simulink model "controllerROS"  (R2021a)
settings: Solver=FixedStepDiscrete  StartTime=0.0  StopTime=200.0  FixedStep=0.02  RelTol=1e-3
undefined symbols (not defined in the file or in its folder): Angular, Linear
libraries: simulink x5, robotlib x3
settings Model: Creator=tian  LastModifiedBy=tian

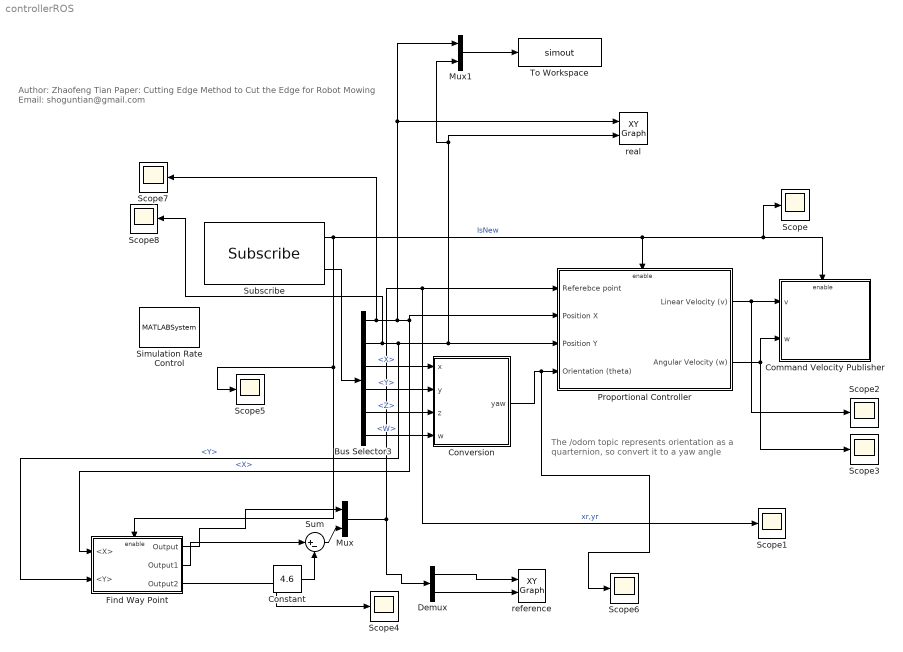
== system controllerROS ==
  note: Author: Zhaofeng Tian
      | Paper: Cutting Edge Method to Cut the Edge for Robot Mowing
      | Email: shoguntian@gmail.com
  note: The /odom topic represents orientation as a quarternion, so convert it to a yaw angle
  Bus Selector3 : BusSelector  OutputSignals=Pose.Pose.Position.X,Pose.Pose.Position.Y,Pose.Pose.Orientation.X,Pose.Pose.Orientation.Y,Pose.Pose.Orientation.Z,Pose.Pose.Orientation.W
  Command Velocity Publisher : Subsystem
  Constant : Constant  Value=4.6
  Conversion : MATLAB Function  TreatAsAtomicUnit=on
  Demux : Demux  Outputs=2
  Find Way Point : Subsystem
  Mux : Mux  Inputs=2
  Mux1 : Mux  Inputs=2
  Proportional Controller : Subsystem
  Scope{,1..8} (9 alike) : Scope
  Simulation Rate Control : MATLABSystem  System=ExampleHelperSimulationRateControl  SampleTime=0.02
      mask Type: ExampleHelperSimulationRateControl
      mask Display: disp('Rate Control');
  Subscribe : robotlib/Subscribe  topicSource=Select from ROS network  topic=/odom  messageType=nav_msgs/Odometry  SampleTime=-1  legacyBusStruct=off  messageQueueLength=51
  Sum : Sum  Inputs=|+-
  To Workspace : ToWorkspace  VariableName=simout  SaveFormat=Timeseries  SampleTime=-1
  real : simulink/Sinks/XY Graph  xmin=-1  xmax=11  ymin=-5  ymax=5  st=-1
  "reference " : simulink/Sinks/XY Graph  xmin=-1  xmax=11  ymin=-5  ymax=5  st=-1
  wires:
  Bus Selector3/2 -> Scope8/1, Find Way Point/2(<Y>), Mux1/2, real/2, Proportional Controller/3(Position Y)  "<Y>"
  Bus Selector3/4 -> Conversion/2(y)  "<Y>"
  Subscribe/1 -> Scope5/1, Find Way Point/Enable, Command Velocity Publisher/Enable, Scope/1, Proportional Controller/Enable  "IsNew"
  Proportional Controller/1(Linear Velocity (v)) -> Scope2/1, Command Velocity Publisher/1(v)
  Bus Selector3/6 -> Conversion/4(w)  "<W>"
  Bus Selector3/1 -> Mux1/1, real/1, Find Way Point/1(<X>), Proportional Controller/2(Position X), Scope7/1  "<X>"
  Mux/1 -> Proportional Controller/1(Referebce point), Scope1/1, Demux/1  "xr,yr"
  Conversion/1(yaw) -> Scope6/1, Proportional Controller/4(Orientation (theta))
  Bus Selector3/5 -> Conversion/3(z)  "<Z>"
  Bus Selector3/3 -> Conversion/1(x)  "<X>"
  Subscribe/2 -> Bus Selector3/1
  Proportional Controller/2(Angular Velocity (w)) -> Command Velocity Publisher/2(w), Scope3/1
  Demux/1 -> "reference "/1
  Demux/2 -> "reference "/2
  Find Way Point/1(Output) -> Mux/1
  Find Way Point/3(Output2) -> Scope4/1
  Mux1/1 -> To Workspace/1
  Find Way Point/2(Output1) -> Sum/1
  Constant/1 -> Sum/2
  Sum/1 -> Mux/2

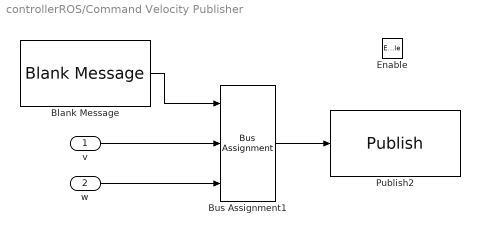
== system controllerROS/Command Velocity Publisher ==
  v : Inport
  w : Inport  Port=2
  Enable : EnablePort
  Blank Message : robotlib/Blank Message  messageClass=Message  entityType=geometry_msgs/Twist  messageType=geometry_msgs/Twist  SampleTime=inf  legacyBusStruct=off
  Bus Assignment1 : BusAssignment  DialogController=Simulink.DDGSource_BusAssignment  AssignedSignals=Linear.X,Angular.Z
  Publish2 : robotlib/Publish  topicSource=Select from ROS network  topic=/cmd_vel  messageType=geometry_msgs/Twist  legacyBusStruct=off  messageQueueLength=105
  wires:
  Bus Assignment1/1 -> Publish2/1
  Blank Message/1 -> Bus Assignment1/1
  v/1 -> Bus Assignment1/2
  w/1 -> Bus Assignment1/3

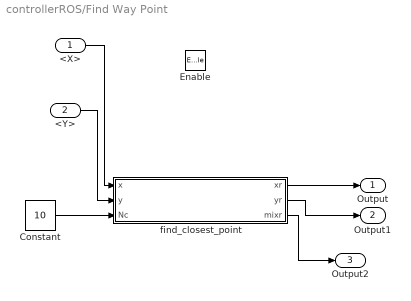
== system controllerROS/Find Way Point ==
  <X> : Inport
  <Y> : Inport  Port=2
  Enable : EnablePort
  Constant : Constant  Value=10
  find_closest_point : MATLAB Function  TreatAsAtomicUnit=on
  Output : Outport
  Output1 : Outport  Port=2
  Output2 : Outport  Port=3
  wires:
  find_closest_point/3(mixr) -> Output2/1
  find_closest_point/2(yr) -> Output1/1
  find_closest_point/1(xr) -> Output/1
  <X>/1 -> find_closest_point/1(x)
  Constant/1 -> find_closest_point/3(Nc)
  <Y>/1 -> find_closest_point/2(y)

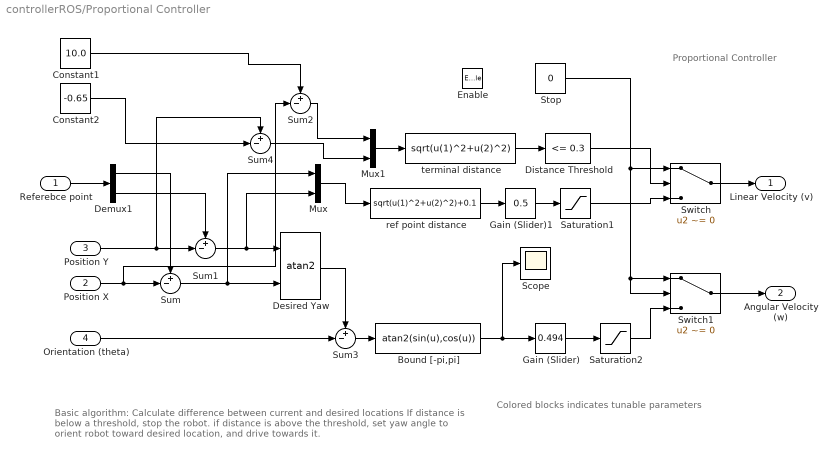
== system controllerROS/Proportional Controller ==
  note: Proportional Controller
  note: Basic algorithm:
      | Calculate difference between current and desired locations
      | If distance is below a threshold, stop the robot.
      | if distance is above the threshold, set yaw angle to orient robot toward desired location, and drive towards it.
  note: Colored blocks indicates tunable parameters
  Referebce point : Inport
  Position X : Inport  Port=2
  Position Y : Inport  Port=3
  Orientation (theta) : Inport  Port=4
  Enable : EnablePort
  Bound [-pi,pi] : Fcn  Expr=atan2(sin(u),cos(u))
  Constant1 : Constant  Value=10.0
  Constant2 : Constant  Value=-0.65
  Demux1 : Demux  Outputs=2
  Desired Yaw : Trigonometry  Operator=atan2
  Distance Threshold : simulink/Logic and Bit Operations/Compare To Constant  relop=<=  const=0.3  OutDataTypeStr=boolean
  Gain (Slider) : simulink/Math Operations/Slider Gain  gain=0.494  low=0.2  high=10
  Gain (Slider)1 : simulink/Math Operations/Slider Gain  gain=0.5  low=0.2  high=10
  Mux : Mux  Inputs=2
  Mux1 : Mux  Inputs=2
  Saturation1 : Saturate  UpperLimit=0.2  LowerLimit=-0.2
  Saturation2 : Saturate  UpperLimit=0.4  LowerLimit=-0.4
  Scope : Scope
  Stop : Constant  Value=0
  Sum{,1..4} (5 alike) : Sum  Inputs=+-|
  Switch : Switch  Criteria=u2 ~= 0
  Switch1 : Switch  Criteria=u2 ~= 0
  ref point distance : Fcn  Expr=sqrt(u(1)^2+u(2)^2)+0.1
  terminal distance : Fcn  Expr=sqrt(u(1)^2+u(2)^2)
  Linear Velocity (v) : Outport  VectorParamsAs1DForOutWhenUnconnected=off
  Angular Velocity (w) : Outport  Port=2  VectorParamsAs1DForOutWhenUnconnected=off
  wires:
  Demux1/1 -> Sum/1
  Demux1/2 -> Sum1/1
  Sum1/1 -> Desired Yaw/1, Mux/2
  Referebce point/1 -> Demux1/1
  Position Y/1 -> Sum4/1, Sum1/2
  Position X/1 -> Sum2/2, Sum/2
  Mux/1 -> ref point distance/1
  Bound [-pi,pi]/1 -> Scope/1, Gain (Slider)/1
  Orientation (theta)/1 -> Sum3/2
  Desired Yaw/1 -> Sum3/1
  Sum/1 -> Desired Yaw/2, Mux/1
  ref point distance/1 -> Gain (Slider)1/1
  Gain (Slider)/1 -> Saturation2/1
  Stop/1 -> Switch/1, Switch1/2, Switch1/1
  Sum3/1 -> Bound [-pi,pi]/1
  Switch/1 -> Linear Velocity (v)/1
  Switch1/1 -> Angular Velocity (w)/1
  Constant1/1 -> Sum2/1
  Constant2/1 -> Sum4/2
  Sum2/1 -> Mux1/1
  Sum4/1 -> Mux1/2
  Mux1/1 -> terminal distance/1
  terminal distance/1 -> Distance Threshold/1
  Distance Threshold/1 -> Switch/2
  Saturation1/1 -> Switch/3
  Saturation2/1 -> Switch1/3
  Gain (Slider)1/1 -> Saturation1/1

== matlab function controllerROS/Conversion ==
  data: yaw output; x input; y input; z input; w input
function yaw  = quat2eul(x,y,z,w)
%#codegen

% Convert the quaternion to a yaw angle (zyx euler angle)
eul = quat2eul([w,x,y,z]);
yaw = eul(1);

end

== matlab function controllerROS/Find Way Point/find_closest_point ==
  data: x input; xr output; y input; Nc input; yr output; mixr output
function [xr,yr,mixr]= find_closest_pont(x,y,Nc)
%load planx and plany
mm =load('roadplan.mat');
planx=mm.nnx*mm.dx;
plany=mm.ylist_line_smooth*mm.dy;
plany=plany';

ixr = ceil(x/mm.dx);% dx = 0.01
if ixr <= 0
    ixr = 1;
end
% Initialization
mind = 1000;
mixr = 1;

% Find min distance loop
if ixr <= 1000-Nc
    for i=ixr:ixr+Nc
        tempd=((planx(i)-x)^2+(plany(i)-y)^2)^0.5;
        if tempd < mind
            mind = tempd;% Update min distance
            mixr = i;         % Update min xr index (ixr)
        end
    end
else
    for i=ixr:1000
        tempd=((planx(i)-x)^2+(plany(i)-y)^2)^0.5;
        if tempd < mind
            mind = tempd;
            mixr = i;
        end
    end
end


xr = planx(mixr);   
yr = plany(mixr);

end
